simulink model "Mixer"  (R2024a)
settings: Solver=ode1be  StartTime=0.0  StopTime=10.0  FixedStep=0.001  RelTol=1e-3
undefined symbols (not defined in the file): cp, M_MIX, mdot_ini, T_ini
settings Model: Creator=ojklem  LastModifiedBy=ojklem

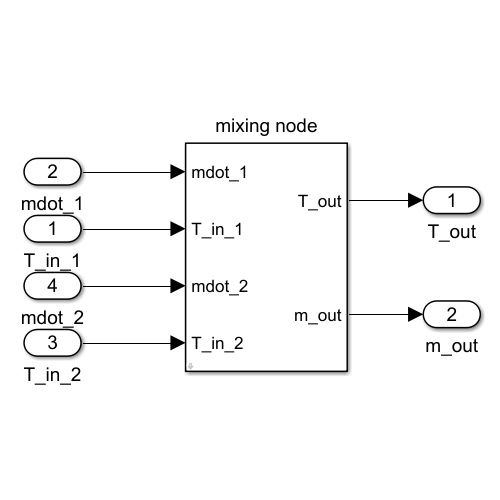
[thumbnail: Simulink's stored preview of the top-level diagram]
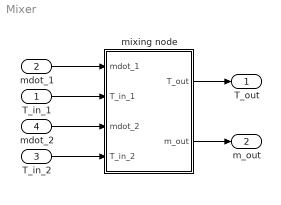
== system Mixer ==
  T_in_1 : Inport
  mdot_1 : Inport  Port=2
  T_in_2 : Inport  Port=3
  mdot_2 : Inport  Port=4
  mixing node : Subsystem  mask{M=M_MIX, cp=cp}
      mask prompts: M "Mass [kg]"; cp "Specific heat capacity [J/kg/K]"
  T_out : Outport
  m_out : Outport  Port=2
  wires:
  mixing node/1(T_out) -> T_out/1
  mixing node/2(m_out) -> m_out/1
  T_in_1/1 -> mixing node/2(T_in_1)
  mdot_1/1 -> mixing node/1(mdot_1)
  T_in_2/1 -> mixing node/4(T_in_2)
  mdot_2/1 -> mixing node/3(mdot_2)

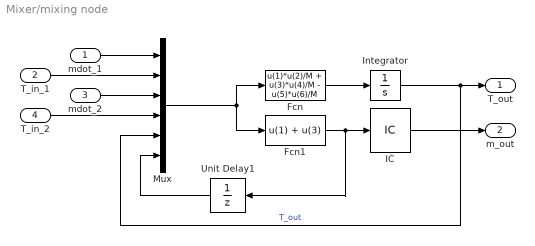
== system Mixer/mixing node ==
  mdot_1 : Inport
  T_in_1 : Inport  Port=2
  mdot_2 : Inport  Port=3
  T_in_2 : Inport  Port=4
  Fcn : Fcn  Expr=u(1)*u(2)/M + u(3)*u(4)/M - u(5)*u(6)/M
  Fcn1 : Fcn  Expr=u(1) + u(3)
  IC : InitialCondition  Value=mdot_ini
  Integrator : Integrator  InitialCondition=T_ini
  Mux : Mux  Inputs=6
  Unit Delay1 : UnitDelay  SampleTime=-1  HasFrameUpgradeWarning=on
  T_out : Outport
  m_out : Outport  Port=2
  wires:
  T_in_2/1 -> Mux/4
  mdot_2/1 -> Mux/3
  T_in_1/1 -> Mux/2
  Fcn/1 -> Integrator/1
  mdot_1/1 -> Mux/1
  Integrator/1 -> Mux/5, T_out/1  "T_out"
  IC/1 -> m_out/1
  Fcn1/1 -> Unit Delay1/1, IC/1
  Mux/1 -> Fcn1/1, Fcn/1
  Unit Delay1/1 -> Mux/6
